simulink model "cruise_model"  (R2020b)
settings: Solver=VariableStepAuto  StartTime=0.0  StopTime=100  RelTol=1e-3
values from neighbouring files (symbols this model uses):
  b = 50.0    [datadic3.sldd]
  Kd = 252.991    [datadic3.sldd]
  Ki = 80.1156    [datadic3.sldd]
  Kp = 471.8559    [datadic3.sldd]
  m = 1000.0    [datadic3.sldd]
settings Model: DataDictionary=datadic3.sldd  Creator=ARPITA  LastModifiedBy=ARPITA
settings DataIOCC: SaveOutput=off  SaveTime=off

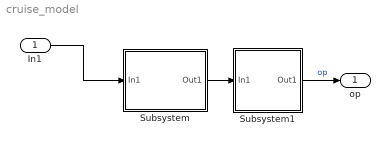
== system cruise_model ==
  In1 : Inport  OutDataTypeStr=double  PortDimensions=1  SampleTime=0
  Subsystem : Subsystem
  Subsystem1 : Subsystem
  op : Outport  OutDataTypeStr=double  PortDimensions=1  SampleTime=0
  wires:
  Subsystem/1(Out1) -> Subsystem1/1(In1)
  Subsystem1/1(Out1) -> op/1  "op"
  In1/1 -> Subsystem/1(In1)

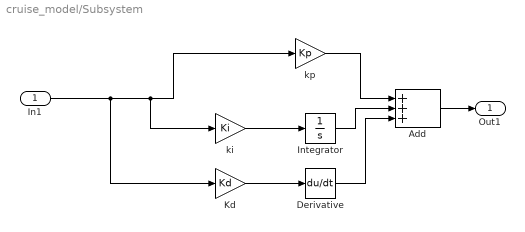
== system cruise_model/Subsystem ==
  In1 : Inport
  Add : Sum  Inputs=+++
  Derivative : Derivative
  Integrator : Integrator
  Kd : Gain  Gain=Kd
  ki : Gain  Gain=Ki
  kp : Gain  Gain=Kp
  Out1 : Outport
  wires:
  Derivative/1 -> Add/3
  Add/1 -> Out1/1
  In1/1 -> Kd/1, ki/1, kp/1
  Integrator/1 -> Add/2
  Kd/1 -> Derivative/1
  ki/1 -> Integrator/1
  kp/1 -> Add/1

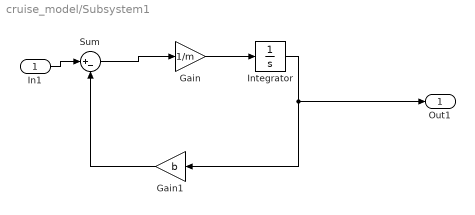
== system cruise_model/Subsystem1 ==
  In1 : Inport
  Gain : Gain  Gain=1/m
  Gain1 : Gain  Gain=b
  Integrator : Integrator
  Sum : Sum  Inputs=|+-
  Out1 : Outport
  wires:
  In1/1 -> Sum/1
  Gain/1 -> Integrator/1
  Sum/1 -> Gain/1
  Gain1/1 -> Sum/2
  Integrator/1 -> Out1/1, Gain1/1
